simulink model "ecp730"  (R2018a)
settings: Solver=ode45  StartTime=0.0  StopTime=5  RelTol=1e-3
libraries: simulink x1
settings Model: Creator=saad  LastModifiedBy=saad
settings SolverCC: ZeroCrossAlgorithm=Adaptive
settings DebuggingCC: MaxConsecutiveZCsMsg=none

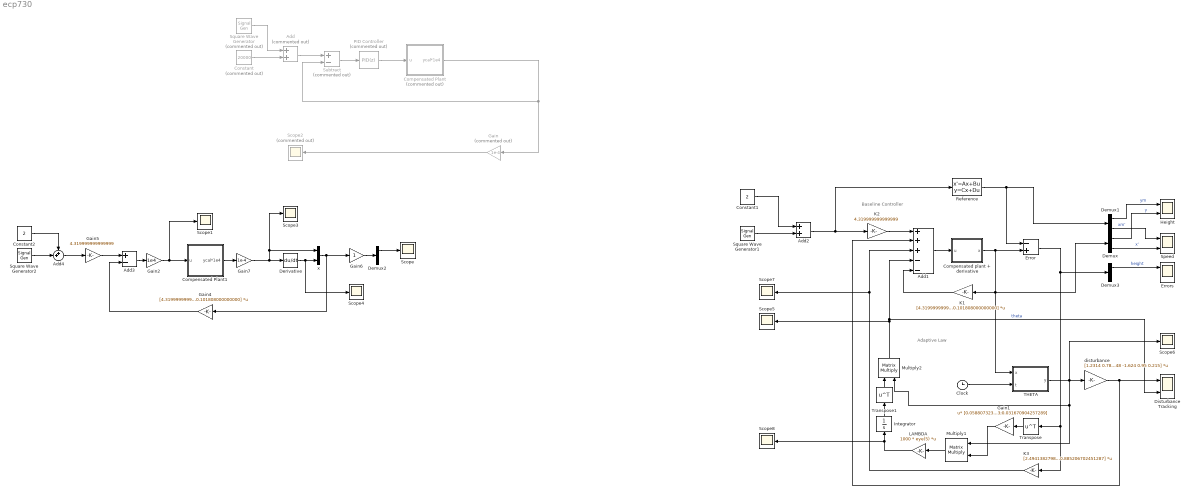
== system ecp730 ==
  note: Baseline Controller
  note: Adaptive Law
  Add : Sum  Commented=on
  Add1 : Sum  Inputs=+++--
  Add2 : Sum
  Add3 : Sum  Inputs=+-
  Add4 : Sum  Inputs=++|
  Clock : Clock
  Compensated Plant : Subsystem  Commented=on
  Compensated Plant1 : Subsystem
  Compensated plant + derivative : Subsystem
  Constant : Constant  Commented=on  Value=20000
  Constant1 : Constant  Value=2
  Constant2 : Constant  Value=2
  Demux{,1..3} (4 alike) : Demux  Outputs=2
  Derivative : Derivative
  Disturbance Tracking : Scope  NumInputPorts=2
  Error : Sum  Inputs=-+
  Errors : Scope  NumInputPorts=2
  Gain : Gain  Commented=on  Gain=1e-4
  Gain1 : Gain  Gain=[0.058807323218383;0.031670904257289]  Multiplication=Matrix(u*K)
  Gain2 : Gain  Gain=1e4
  Gain4 : Gain  Gain=[4.319999999999999,0.101808000000000]  Multiplication=Matrix(K*u)
  Gain5 : Gain  Gain=4.319999999999999
  Gain6 : Gain
  Gain7 : Gain  Gain=1e-4
  Height : Scope  NumInputPorts=2
  Integrator : Integrator
  K1 : Gain  Gain=[4.319999999999999,0.101808000000000]  Multiplication=Matrix(K*u)
  K2 : Gain  Gain=4.319999999999999
  K3 : Gain  Gain=[2.494138279869975,-0.885206702451287]  Multiplication=Matrix(K*u)
  LAMBDA : Gain  Gain=1000 * eye(5)  Multiplication=Matrix(K*u)
  Multiply1 : Product  Multiplication=Matrix(*)
  Multiply2 : Product  Multiplication=Matrix(*)
  PID Controller : simulink/Continuous/PID Controller  Commented=on  Controller=PID  TimeDomain=Discrete-time  SampleTime=0.001768  IntegratorMethod=Forward Euler  FilterMethod=Forward Euler  Form=Parallel  UseFilter=on  ControllerParametersSource=internal  P=1.65  I=0  D=0.065  N=100  InitialConditionSource=internal  InitialConditionForIntegrator=0  InitialConditionForFilter=0  ExternalReset=none  LimitOutput=off  UpperSaturationLimit=inf  LowerSaturationLimit=-inf  LinearizeAsGain=on  AntiWindupMode=none  Kb=1  TrackingMode=off  Kt=1  PParamMin=[]  PParamMax=[]  IParamMin=[]  IParamMax=[]  DParamMin=[]  DParamMax=[]  NParamMin=[]  NParamMax=[]  KbParamMin=[]  KbParamMax=[]  KtParamMin=[]  KtParamMax=[]  POutMin=[]  POutMax=[]  IOutMin=[]  IOutMax=[]  DOutMin=[]  DOutMax=[]  NOutMin=[]  NOutMax=[]  KbOutMin=[]  KbOutMax=[]  KtOutMin=[]  KtOutMax=[]  IntegratorOutMin=[]  IntegratorOutMax=[]  FilterOutMin=[]  FilterOutMax=[]  SumOutMin=[]  SumOutMax=[]  SumI1OutMin=[]  SumI1OutMax=[]  SumI2OutMin=[]  SumI2OutMax=[]  SumI3OutMin=[]  SumI3OutMax=[]  SumDOutMin=[]  SumDOutMax=[]  SaturationOutMin=[]  SaturationOutMax=[]  IntegratorContinuousStateAttributes=''  IntegratorStateMustResolveToSignalObject=off  IntegratorRTWStateStorageClass=Auto  FilterContinuousStateAttributes=''  FilterStateMustResolveToSignalObject=off  FilterRTWStateStorageClass=Auto  DifferentiatorICPrevScaledInput=0  DifferentiatorOutMin=[]  DifferentiatorOutMax=[]  FilterDiffOutCoefMin=[]  FilterDiffOutCoefMax=[]  SumDenOutMin=[]  SumDenOutMax=[]  SumNumOutMin=[]  SumNumOutMax=[]  ReciprocalOutMin=[]  ReciprocalOutMax=[]  DivideOutMin=[]  DivideOutMax=[]  TunerSelectOption=Transfer Function Based (PID Tuner App)
  Reference : StateSpace  A=[0,1;-3600,-84.839999999999990]  B=[0;3600]  C=eye(2)  D=[0;0]  InitialCondition=0  ContinuousStateAttributes={'angle', 'angular_speed'}
  Scope{,1,3..8} (8 alike) : Scope
  Scope2 : Scope  Commented=on
  Speed : Scope  NumInputPorts=2
  Square Wave Generator : SignalGenerator  Commented=on  WaveForm=square  Amplitude=5000
  Square Wave Generator1 : SignalGenerator  WaveForm=square  Amplitude=0.5
  Square Wave Generator2 : SignalGenerator  WaveForm=square  Amplitude=0.5
  Subtract : Sum  Commented=on  Inputs=+-
  THETA : MATLAB Function  TreatAsAtomicUnit=on
  Transpose : Math  Operator=transpose  SaturateOnIntegerOverflow=on
  Transpose1 : Math  Operator=transpose  SaturateOnIntegerOverflow=on
  disturbance : Gain  Gain=[1.2314 0.7848 -1.624 0.95 0.215]  Multiplication=Matrix(K*u)
  x : Mux  Inputs=2
  wires:
  Gain/1 -> Scope2/1
  Compensated Plant/1(ycal*1e4) -> Subtract/2, Gain/1
  PID Controller/1 -> Compensated Plant/1(u)
  Subtract/1 -> PID Controller/1
  Add/1 -> Subtract/1
  Constant/1 -> Add/2
  Square Wave Generator/1 -> Add/1
  Compensated plant + derivative/1(x) -> Error/2, THETA/1(x), Demux/1, K1/1
  Reference/1 -> Error/1, Demux1/1
  THETA/1(y) -> disturbance/1, Scope6/1, Multiply2/2, Multiply1/1
  disturbance/1 -> Add1/2, Disturbance Tracking/1
  Integrator/1 -> Transpose1/1
  K1/1 -> Add1/5
  Demux1/2 -> Speed/1  "xm'"
  K2/1 -> Add1/1
  LAMBDA/1 -> Scope8/1, Integrator/1
  Demux3/1 -> Errors/1  "height"
  Demux1/1 -> Height/1  "ym"
  Error/1 -> Demux3/1, K3/1, Transpose/1
  Add1/1 -> Compensated plant + derivative/1(u)
  Demux/1 -> Height/2  "y"
  Transpose1/1 -> Multiply2/1
  Demux/2 -> Speed/2  "x'"
  Multiply1/1 -> LAMBDA/1
  Gain1/1 -> Multiply1/2
  Transpose/1 -> Gain1/1
  Constant1/1 -> Add2/1
  Square Wave Generator1/1 -> Add2/2
  Add2/1 -> Reference/1, K2/1
  Derivative/1 -> Scope4/1, x/2
  x/1 -> Gain6/1, Gain4/1
  Add3/1 -> Gain2/1
  Gain4/1 -> Add3/2
  Gain5/1 -> Add3/1
  Add4/1 -> Gain5/1
  Square Wave Generator2/1 -> Add4/2
  Constant2/1 -> Add4/1
  Gain6/1 -> Demux2/1
  Demux2/1 -> Scope/1
  Compensated Plant1/1(ycal*1e4) -> Gain7/1
  Gain7/1 -> Scope3/1, x/1, Derivative/1
  Multiply2/1 -> Add1/4, Disturbance Tracking/2, Scope5/1  "theta"
  K3/1 -> Add1/3, Scope7/1
  Gain2/1 -> Scope1/1, Compensated Plant1/1(u)
  Clock/1 -> THETA/2(t)

== system ecp730/Compensated Plant ==
  u : Inport
  Add : Sum  Inputs=++|
  Gravity Correction : Constant  Value=11760
  Nonlinear Plant : Subsystem
  Nonlinearity Compensation : Subsystem
  Scope1 : Scope
  Sensor Nonlinearity Correction : Subsystem
  ycal*1e4 : Outport
  wires:
  Nonlinearity Compensation/1(u*) -> Scope1/1, Nonlinear Plant/1(u)
  Add/1 -> Nonlinearity Compensation/1(u)
  Gravity Correction/1 -> Add/1
  Sensor Nonlinearity Correction/1("ycal*1e4 ") -> ycal*1e4/1, Nonlinearity Compensation/2(ycal*1e4)
  u/1 -> Add/2
  Nonlinear Plant/1(Sensor (yraw)) -> Sensor Nonlinearity Correction/1(yraw (counts))

== system ecp730/Compensated Plant1 ==
  u : Inport
  Add : Sum  Inputs=++|
  Gravity Correction : Constant  Value=11760
  Nonlinear Plant : Subsystem
  Nonlinearity Compensation : Subsystem
  Saturation : Saturate  UpperLimit=30000  LowerLimit=-30000
  Scope1 : Scope
  Scope2 : Scope
  Sensor Nonlinearity Correction : Subsystem
  ycal*1e4 : Outport
  wires:
  Nonlinearity Compensation/1(u*) -> Scope1/1, Nonlinear Plant/1(u)
  Add/1 -> Saturation/1
  Gravity Correction/1 -> Add/1
  Sensor Nonlinearity Correction/1("ycal*1e4 ") -> ycal*1e4/1, Nonlinearity Compensation/2(ycal*1e4)
  u/1 -> Add/2
  Nonlinear Plant/1(Sensor (yraw)) -> Sensor Nonlinearity Correction/1(yraw (counts))
  Saturation/1 -> Scope2/1, Nonlinearity Compensation/1(u)

== system ecp730/Compensated plant + derivative ==
  u : Inport
  Compensated Plant1 : Subsystem
  Derivative : Derivative
  Gain : Gain  Gain=1e-4
  Gain1 : Gain  Gain=1e4
  Mux : Mux  Inputs=2
  Scope : Scope
  Scope1 : Scope
  x : Outport
  wires:
  Mux/1 -> x/1
  Derivative/1 -> Scope/1, Mux/2
  Compensated Plant1/1(ycal*1e4) -> Gain/1
  Gain/1 -> Mux/1, Derivative/1
  u/1 -> Gain1/1
  Gain1/1 -> Scope1/1, Compensated Plant1/1(u)

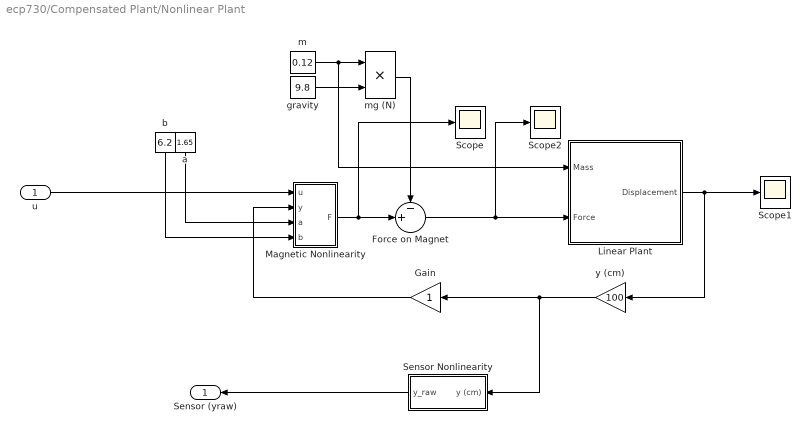
== system ecp730/Compensated Plant/Nonlinear Plant ==
  u : Inport
  Force on Magnet : Sum  Inputs=-+|
  Gain : Gain
  Linear Plant : Subsystem
  Magnetic Nonlinearity : Subsystem
  Scope : Scope
  Scope1 : Scope
  Scope2 : Scope
  Sensor Nonlinearity : Subsystem
  a : Constant  Value=1.65
  b : Constant  Value=6.2
  gravity : Constant  Value=9.8
  m : Constant  Value=0.12
  mg (N) : Product
  y (cm) : Gain  Gain=100
  Sensor (yraw) : Outport
  wires:
  Magnetic Nonlinearity/1(F) -> Scope/1, Force on Magnet/2
  u/1 -> Magnetic Nonlinearity/1(u)
  Force on Magnet/1 -> Scope2/1, Linear Plant/2(Force)
  y (cm)/1 -> Sensor Nonlinearity/1(y (cm)), Gain/1
  b/1 -> Magnetic Nonlinearity/4(b)
  mg (N)/1 -> Force on Magnet/1
  m/1 -> mg (N)/1, Linear Plant/1(Mass)
  Sensor Nonlinearity/1(y_raw) -> Sensor (yraw)/1
  a/1 -> Magnetic Nonlinearity/3(a)
  gravity/1 -> mg (N)/2
  Linear Plant/1(Displacement) -> Scope1/1, y (cm)/1
  Gain/1 -> Magnetic Nonlinearity/2(y)

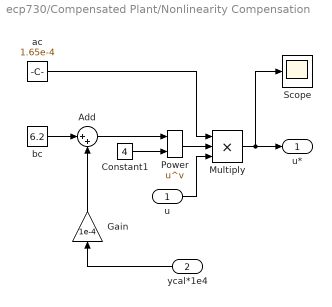
== system ecp730/Compensated Plant/Nonlinearity Compensation ==
  u : Inport
  ycal*1e4 : Inport  Port=2
  Add : Sum  Inputs=|++
  Constant1 : Constant  Value=4
  Gain : Gain  Gain=1e-4
  Multiply : Product  Inputs=3
  Power : Math  Operator=pow  SaturateOnIntegerOverflow=on
  Scope : Scope
  ac : Constant  Value=1.65e-4
  bc : Constant  Value=6.2
  u* : Outport
  wires:
  Constant1/1 -> Power/2
  ac/1 -> Multiply/1
  bc/1 -> Add/1
  ycal*1e4/1 -> Gain/1
  Power/1 -> Multiply/2
  Gain/1 -> Add/2
  Add/1 -> Power/1
  u/1 -> Multiply/3
  Multiply/1 -> Scope/1, u*/1

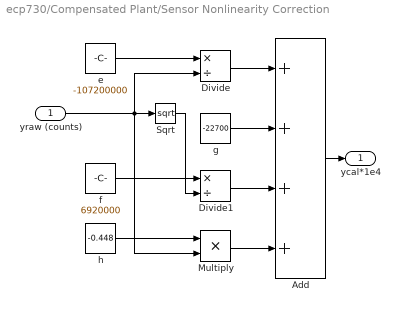
== system ecp730/Compensated Plant/Sensor Nonlinearity Correction ==
  yraw (counts) : Inport
  Add : Sum  Inputs=++++
  Divide : Product  Inputs=*/
  Divide1 : Product  Inputs=*/
  Multiply : Product
  Sqrt : Sqrt  SaturateOnIntegerOverflow=on
  e : Constant  Value=-107200000
  f : Constant  Value=6920000
  g : Constant  Value=-22700
  h : Constant  Value=-0.448
  "ycal*1e4 " : Outport
  wires:
  g/1 -> Add/2
  Add/1 -> "ycal*1e4 "/1
  h/1 -> Multiply/1
  Divide1/1 -> Add/3
  yraw (counts)/1 -> Multiply/2, Sqrt/1, Divide/2
  Multiply/1 -> Add/4
  e/1 -> Divide/1
  Divide/1 -> Add/1
  f/1 -> Divide1/1
  Sqrt/1 -> Divide1/2

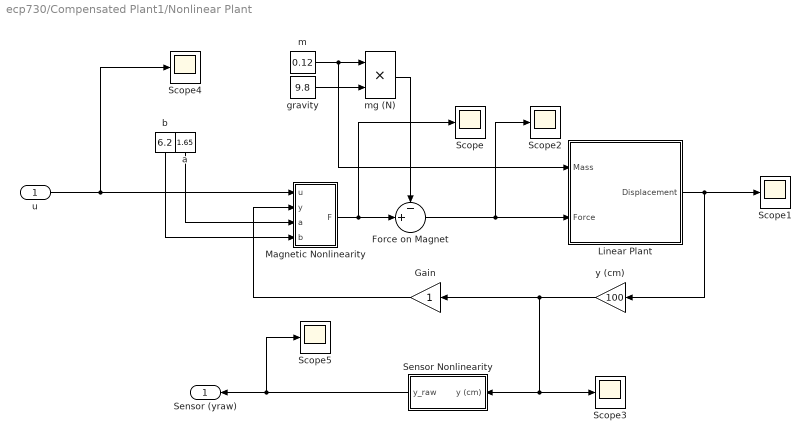
== system ecp730/Compensated Plant1/Nonlinear Plant ==
  u : Inport
  Force on Magnet : Sum  Inputs=-+|
  Gain : Gain
  Linear Plant : Subsystem
  Magnetic Nonlinearity : Subsystem
  Scope{,1..5} (6 alike) : Scope
  Sensor Nonlinearity : Subsystem
  a : Constant  Value=1.65
  b : Constant  Value=6.2
  gravity : Constant  Value=9.8
  m : Constant  Value=0.12
  mg (N) : Product
  y (cm) : Gain  Gain=100
  Sensor (yraw) : Outport
  wires:
  Magnetic Nonlinearity/1(F) -> Scope/1, Force on Magnet/2
  u/1 -> Scope4/1, Magnetic Nonlinearity/1(u)
  Force on Magnet/1 -> Scope2/1, Linear Plant/2(Force)
  y (cm)/1 -> Sensor Nonlinearity/1(y (cm)), Scope3/1, Gain/1
  b/1 -> Magnetic Nonlinearity/4(b)
  mg (N)/1 -> Force on Magnet/1
  m/1 -> mg (N)/1, Linear Plant/1(Mass)
  Sensor Nonlinearity/1(y_raw) -> Scope5/1, Sensor (yraw)/1
  a/1 -> Magnetic Nonlinearity/3(a)
  gravity/1 -> mg (N)/2
  Linear Plant/1(Displacement) -> Scope1/1, y (cm)/1
  Gain/1 -> Magnetic Nonlinearity/2(y)

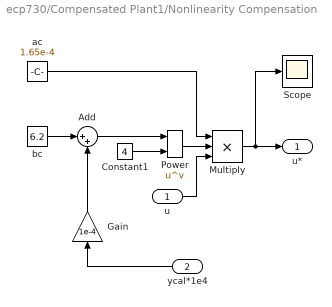
== system ecp730/Compensated Plant1/Nonlinearity Compensation ==
  u : Inport
  ycal*1e4 : Inport  Port=2
  Add : Sum  Inputs=|++
  Constant1 : Constant  Value=4
  Gain : Gain  Gain=1e-4
  Multiply : Product  Inputs=3
  Power : Math  Operator=pow  SaturateOnIntegerOverflow=on
  Scope : Scope
  ac : Constant  Value=1.65e-4
  bc : Constant  Value=6.2
  u* : Outport
  wires:
  Constant1/1 -> Power/2
  ac/1 -> Multiply/1
  bc/1 -> Add/1
  ycal*1e4/1 -> Gain/1
  Power/1 -> Multiply/2
  Gain/1 -> Add/2
  Add/1 -> Power/1
  u/1 -> Multiply/3
  Multiply/1 -> Scope/1, u*/1

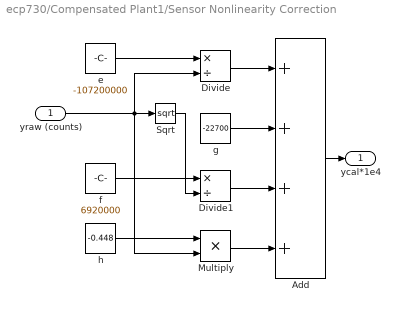
== system ecp730/Compensated Plant1/Sensor Nonlinearity Correction ==
  yraw (counts) : Inport
  Add : Sum  Inputs=++++
  Divide : Product  Inputs=*/
  Divide1 : Product  Inputs=*/
  Multiply : Product
  Sqrt : Sqrt  SaturateOnIntegerOverflow=on
  e : Constant  Value=-107200000
  f : Constant  Value=6920000
  g : Constant  Value=-22700
  h : Constant  Value=-0.448
  "ycal*1e4 " : Outport
  wires:
  g/1 -> Add/2
  Add/1 -> "ycal*1e4 "/1
  h/1 -> Multiply/1
  Divide1/1 -> Add/3
  yraw (counts)/1 -> Multiply/2, Sqrt/1, Divide/2
  Multiply/1 -> Add/4
  e/1 -> Divide/1
  Divide/1 -> Add/1
  f/1 -> Divide1/1
  Sqrt/1 -> Divide1/2

== system ecp730/Compensated plant + derivative/Compensated Plant1 ==
  u : Inport
  Add : Sum  Inputs=++|
  Gravity Correction : Constant  Value=11760
  Nonlinear Plant : Subsystem
  Nonlinearity Compensation : Subsystem
  Saturation : Saturate  UpperLimit=30000  LowerLimit=-30000  ZeroCross=off
  Scope1 : Scope
  Sensor Nonlinearity Correction : Subsystem
  ycal*1e4 : Outport
  wires:
  Nonlinearity Compensation/1(u*) -> Saturation/1
  Gravity Correction/1 -> Add/1
  Sensor Nonlinearity Correction/1("ycal*1e4 ") -> ycal*1e4/1, Nonlinearity Compensation/2(ycal*1e4)
  u/1 -> Add/2
  Nonlinear Plant/1(Sensor (yraw)) -> Sensor Nonlinearity Correction/1(yraw (counts))
  Add/1 -> Nonlinearity Compensation/1(u)
  Saturation/1 -> Scope1/1, Nonlinear Plant/1(u)

== system ecp730/Compensated Plant/Nonlinear Plant/Linear Plant ==
  Mass : Inport
  Force : Inport  Port=2
  "Acceleration " : Product  Inputs=/*
  "Displacement " : Integrator  LowerSaturationLimit=0
  Scope : Scope
  Scope1 : Scope
  Scope2 : Scope
  "Velocity " : Integrator
  Displacement : Outport
  wires:
  Force/1 -> "Acceleration "/2
  Mass/1 -> "Acceleration "/1
  "Displacement "/1 -> Scope2/1, Displacement/1
  "Velocity "/1 -> Scope1/1, "Displacement "/1
  "Acceleration "/1 -> Scope/1, "Velocity "/1

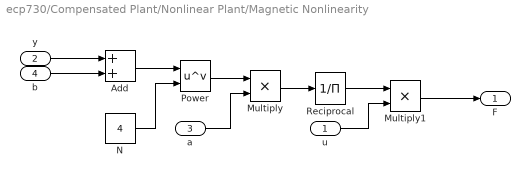
== system ecp730/Compensated Plant/Nonlinear Plant/Magnetic Nonlinearity ==
  u : Inport
  y : Inport  Port=2
  a : Inport  Port=3
  b : Inport  Port=4
  Add : Sum
  Multiply : Product
  Multiply1 : Product
  N : Constant  Value=4
  Power : Math  Operator=pow  SaturateOnIntegerOverflow=on
  Reciprocal : Product  Inputs=/
  F : Outport
  wires:
  y/1 -> Add/1
  a/1 -> Multiply/2
  Add/1 -> Power/1
  N/1 -> Power/2
  u/1 -> Multiply1/2
  Power/1 -> Multiply/1
  Multiply/1 -> Reciprocal/1
  b/1 -> Add/2
  Multiply1/1 -> F/1
  Reciprocal/1 -> Multiply1/1

== system ecp730/Compensated Plant/Nonlinear Plant/Sensor Nonlinearity ==
  y (cm) : Inport
  Constant1 : Constant  Value=-0.3504
  Constant2 : Constant  Value=3.029e+04
  Exp : Math  SaturateOnIntegerOverflow=on
  Multiply : Product
  Multiply1 : Product
  y_raw : Outport
  wires:
  Constant2/1 -> Multiply1/2
  Exp/1 -> Multiply1/1
  Multiply1/1 -> y_raw/1
  y (cm)/1 -> Multiply/2
  Constant1/1 -> Multiply/1
  Multiply/1 -> Exp/1

== system ecp730/Compensated Plant1/Nonlinear Plant/Linear Plant ==
  Mass : Inport
  Force : Inport  Port=2
  "Acceleration " : Product  Inputs=/*
  "Displacement " : Integrator  LowerSaturationLimit=0
  Scope : Scope
  Scope1 : Scope
  Scope2 : Scope
  "Velocity " : Integrator
  Displacement : Outport
  wires:
  Force/1 -> "Acceleration "/2
  Mass/1 -> "Acceleration "/1
  "Displacement "/1 -> Scope2/1, Displacement/1
  "Velocity "/1 -> Scope1/1, "Displacement "/1
  "Acceleration "/1 -> Scope/1, "Velocity "/1

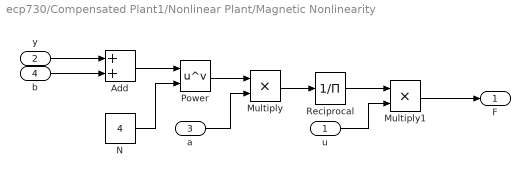
== system ecp730/Compensated Plant1/Nonlinear Plant/Magnetic Nonlinearity ==
  u : Inport
  y : Inport  Port=2
  a : Inport  Port=3
  b : Inport  Port=4
  Add : Sum
  Multiply : Product
  Multiply1 : Product
  N : Constant  Value=4
  Power : Math  Operator=pow  SaturateOnIntegerOverflow=on
  Reciprocal : Product  Inputs=/
  F : Outport
  wires:
  y/1 -> Add/1
  a/1 -> Multiply/2
  Add/1 -> Power/1
  N/1 -> Power/2
  u/1 -> Multiply1/2
  Power/1 -> Multiply/1
  Multiply/1 -> Reciprocal/1
  b/1 -> Add/2
  Multiply1/1 -> F/1
  Reciprocal/1 -> Multiply1/1

== system ecp730/Compensated Plant1/Nonlinear Plant/Sensor Nonlinearity ==
  y (cm) : Inport
  Constant1 : Constant  Value=-0.3504
  Constant2 : Constant  Value=3.029e+04
  Exp : Math  SaturateOnIntegerOverflow=on
  Multiply : Product
  Multiply1 : Product
  y_raw : Outport
  wires:
  Constant2/1 -> Multiply1/2
  Exp/1 -> Multiply1/1
  Multiply1/1 -> y_raw/1
  y (cm)/1 -> Multiply/2
  Constant1/1 -> Multiply/1
  Multiply/1 -> Exp/1

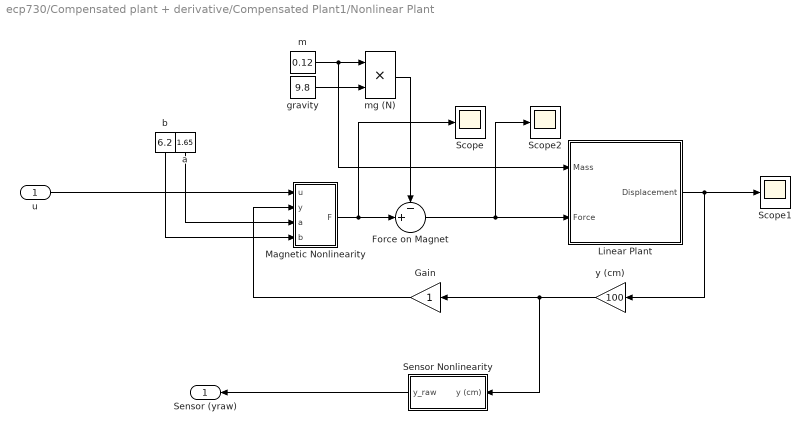
== system ecp730/Compensated plant + derivative/Compensated Plant1/Nonlinear Plant ==
  u : Inport
  Force on Magnet : Sum  Inputs=-+|
  Gain : Gain
  Linear Plant : Subsystem
  Magnetic Nonlinearity : Subsystem
  Scope : Scope
  Scope1 : Scope
  Scope2 : Scope
  Sensor Nonlinearity : Subsystem
  a : Constant  Value=1.65
  b : Constant  Value=6.2
  gravity : Constant  Value=9.8
  m : Constant  Value=0.12
  mg (N) : Product
  y (cm) : Gain  Gain=100
  Sensor (yraw) : Outport
  wires:
  Magnetic Nonlinearity/1(F) -> Scope/1, Force on Magnet/2
  u/1 -> Magnetic Nonlinearity/1(u)
  Force on Magnet/1 -> Scope2/1, Linear Plant/2(Force)
  y (cm)/1 -> Sensor Nonlinearity/1(y (cm)), Gain/1
  b/1 -> Magnetic Nonlinearity/4(b)
  mg (N)/1 -> Force on Magnet/1
  m/1 -> mg (N)/1, Linear Plant/1(Mass)
  Sensor Nonlinearity/1(y_raw) -> Sensor (yraw)/1
  a/1 -> Magnetic Nonlinearity/3(a)
  gravity/1 -> mg (N)/2
  Linear Plant/1(Displacement) -> Scope1/1, y (cm)/1
  Gain/1 -> Magnetic Nonlinearity/2(y)

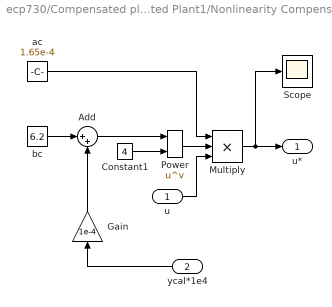
== system ecp730/Compensated plant + derivative/Compensated Plant1/Nonlinearity Compensation ==
  u : Inport
  ycal*1e4 : Inport  Port=2
  Add : Sum  Inputs=|++
  Constant1 : Constant  Value=4
  Gain : Gain  Gain=1e-4
  Multiply : Product  Inputs=3
  Power : Math  Operator=pow  SaturateOnIntegerOverflow=on
  Scope : Scope
  ac : Constant  Value=1.65e-4
  bc : Constant  Value=6.2
  u* : Outport
  wires:
  Constant1/1 -> Power/2
  ac/1 -> Multiply/1
  bc/1 -> Add/1
  ycal*1e4/1 -> Gain/1
  Power/1 -> Multiply/2
  Gain/1 -> Add/2
  Add/1 -> Power/1
  u/1 -> Multiply/3
  Multiply/1 -> Scope/1, u*/1

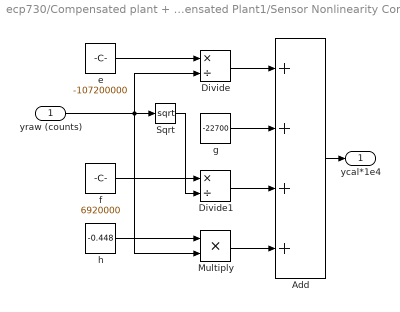
== system ecp730/Compensated plant + derivative/Compensated Plant1/Sensor Nonlinearity Correction ==
  yraw (counts) : Inport
  Add : Sum  Inputs=++++
  Divide : Product  Inputs=*/
  Divide1 : Product  Inputs=*/
  Multiply : Product
  Sqrt : Sqrt  SaturateOnIntegerOverflow=on
  e : Constant  Value=-107200000
  f : Constant  Value=6920000
  g : Constant  Value=-22700
  h : Constant  Value=-0.448
  "ycal*1e4 " : Outport
  wires:
  g/1 -> Add/2
  Add/1 -> "ycal*1e4 "/1
  h/1 -> Multiply/1
  Divide1/1 -> Add/3
  yraw (counts)/1 -> Multiply/2, Sqrt/1, Divide/2
  Multiply/1 -> Add/4
  e/1 -> Divide/1
  Divide/1 -> Add/1
  f/1 -> Divide1/1
  Sqrt/1 -> Divide1/2

== system ecp730/Compensated plant + derivative/Compensated Plant1/Nonlinear Plant/Linear Plant ==
  Mass : Inport
  Force : Inport  Port=2
  "Acceleration " : Product  Inputs=/*
  "Displacement " : Integrator  LowerSaturationLimit=0
  Scope : Scope
  Scope1 : Scope
  Scope2 : Scope
  "Velocity " : Integrator
  Displacement : Outport
  wires:
  Force/1 -> "Acceleration "/2
  Mass/1 -> "Acceleration "/1
  "Displacement "/1 -> Scope2/1, Displacement/1
  "Velocity "/1 -> Scope1/1, "Displacement "/1
  "Acceleration "/1 -> Scope/1, "Velocity "/1

== system ecp730/Compensated plant + derivative/Compensated Plant1/Nonlinear Plant/Magnetic Nonlinearity ==
  u : Inport
  y : Inport  Port=2
  a : Inport  Port=3
  b : Inport  Port=4
  Add : Sum
  Multiply : Product
  Multiply1 : Product
  N : Constant  Value=4
  Power : Math  Operator=pow  SaturateOnIntegerOverflow=on
  Reciprocal : Product  Inputs=/
  F : Outport
  wires:
  y/1 -> Add/1
  a/1 -> Multiply/2
  Add/1 -> Power/1
  N/1 -> Power/2
  u/1 -> Multiply1/2
  Power/1 -> Multiply/1
  Multiply/1 -> Reciprocal/1
  b/1 -> Add/2
  Multiply1/1 -> F/1
  Reciprocal/1 -> Multiply1/1

== system ecp730/Compensated plant + derivative/Compensated Plant1/Nonlinear Plant/Sensor Nonlinearity ==
  y (cm) : Inport
  Constant1 : Constant  Value=-0.3504
  Constant2 : Constant  Value=3.029e+04
  Exp : Math  SaturateOnIntegerOverflow=on
  Multiply : Product
  Multiply1 : Product
  y_raw : Outport
  wires:
  Constant2/1 -> Multiply1/2
  Exp/1 -> Multiply1/1
  Multiply1/1 -> y_raw/1
  y (cm)/1 -> Multiply/2
  Constant1/1 -> Multiply/1
  Multiply/1 -> Exp/1

== matlab function ecp730/THETA ==
  data: x input; y output; t input
function y = fcn(x,t)

    %y = [x(1); x(2); abs(x(1))*x(2); abs(x(2))*x(2); x(1)^3];
    %y = [x(1)^2; x(1) > 0; sin(x(1)); cos(x(1)); x(1)];
    y = [x(1); 0; sin(2*pi*t); 0; 0];
